simulink model "sim_battery"  (R2022b)
settings: Solver=VariableStepAuto  StartTime=0.0  StopTime=2001  RelTol=1e-3
undefined symbols (not defined in the file or in its folder): battery_builder_rtmsupport, gcbh
libraries: nesl_utility x14, GD_Batterymodel_5_lib x8, fl_lib x7, BatteryCurrentManagement x1, batt_lib x1, BatteryBalancing x1, simulink x1, SimscapeFluids_lib x1
(part 2 of 2)

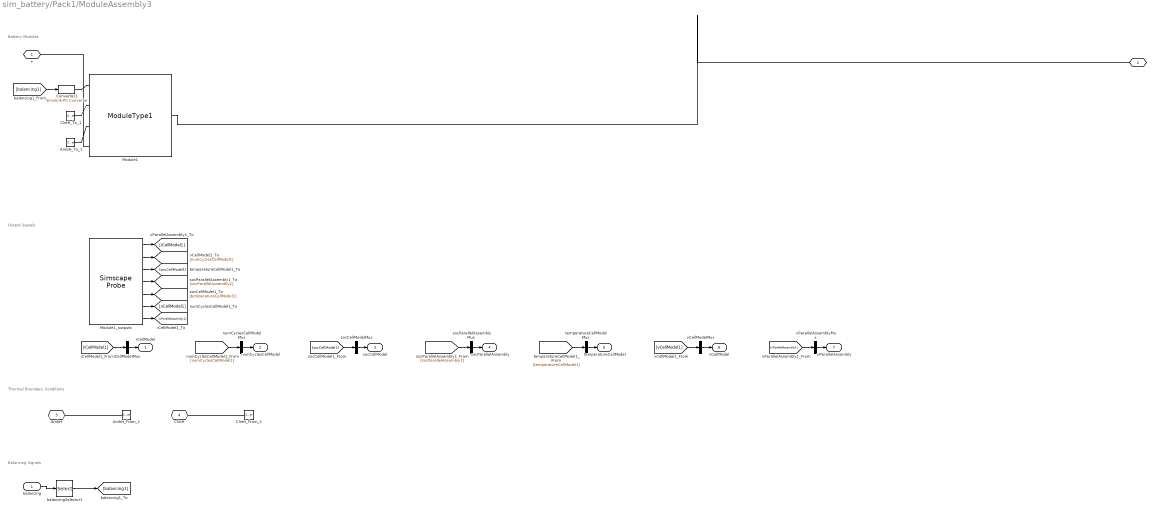
== system sim_battery/Pack1/ModuleAssembly3 ==
  note: Balancing Signals
  note: Thermal Boundary Conditions
  note: Output Signals
  note: Battery Modules
  balancing : Inport  PortDimensions=14
  AmbH_From_1 : ConnectionLabel  Label=ambH_1
  AmbH_To_1 : ConnectionLabel  Label=ambH_1
  ClntH_From_1 : ConnectionLabel  Label=clntH_1
  ClntH_To_1 : ConnectionLabel  Label=clntH_1
  Converter1 : nesl_utility/Simulink-PS Converter  PhysicalDomain=network_engine_domain  SubClassName=ps_input  LeftPortType=input  RightPortType=output  PseudoPeriodic=off  Frequencies=[]  NoiseDistribution=none  NoiseParameters=[]  Unit=1  AffineConversion=off  FilteringAndDerivatives=provide  SimscapeFilterOrder=1  InputFilterTimeConstant=0.001  UdotUserProvided=0
  Module1 : GD_Batterymodel_5_lib/Modules/ModuleType1  SOC_vec=ModuleType1.SOC_vec  T_vec=ModuleType1.T_vec K  V0_mat=ModuleType1.V0_mat V  V_range=ModuleType1.V_range V  R0_mat=ModuleType1.R0_mat Ohm  AH=ModuleType1.AH A*hr  extrapolation_option=simscape.enum.extrapolation.nearest  R1_mat=ModuleType1.R1_mat Ohm  tau1_mat=ModuleType1.tau1_mat s  R2_mat=ModuleType1.R2_mat Ohm  tau2_mat=ModuleType1.tau2_mat s  thermal_mass=ModuleType1.thermal_mass J/K  CoolantResistance=ModuleType1.CoolantResistance K/W  AmbientResistance=ModuleType1.AmbientResistance K/W  CellBalancingClosedResistance=ModuleType1.CellBalancingClosedResistance Ohm  CellBalancingOpenConductance=ModuleType1.CellBalancingOpenConductance 1/Ohm  CellBalancingThreshold=ModuleType1.CellBalancingThreshold  CellBalancingResistance=ModuleType1.CellBalancingResistance Ohm  P=3  S=14  iCellModel_specify=on  iCellModel_priority=None  iCellModel=ModuleAssembly3.Module1.iCellModel A  iCellModel_nominal_specify=off  iCellModel_nominal_unit=A  iCellModel_nominal_value=1  vCellModel_specify=on  vCellModel_priority=None  vCellModel=ModuleAssembly3.Module1.vCellModel V  vCellModel_nominal_specify=off  vCellModel_nominal_unit=V  vCellModel_nominal_value=1  socCellModel_specify=on  socCellModel_priority=High  socCellModel=ModuleAssembly3.Module1.socCellModel  socCellModel_nominal_specify=off  socCellModel_nominal_unit=1  socCellModel_nominal_value=1  numCyclesCellModel_specify=on  numCyclesCellModel_priority=High  numCyclesCellModel=ModuleAssembly3.Module1.numCyclesCellModel  numCyclesCellModel_nominal_specify=off  numCyclesCellModel_nominal_unit=1  numCyclesCellModel_nominal_value=1  temperatureCellModel_specify=on  temperatureCellModel_priority=High  temperatureCellModel=ModuleAssembly3.Module1.temperatureCellModel K  temperatureCellModel_nominal_specify=off  temperatureCellModel_nominal_unit=K  temperatureCellModel_nominal_value=1  vParallelAssembly_specify=on  vParallelAssembly_priority=None  vParallelAssembly=ModuleAssembly3.Module1.vParallelAssembly V  vParallelAssembly_nominal_specify=off  vParallelAssembly_nominal_unit=V  vParallelAssembly_nominal_value=1  socParallelAssembly_specify=on  socParallelAssembly_priority=None  socParallelAssembly=ModuleAssembly3.Module1.socParallelAssembly  socParallelAssembly_nominal_specify=off  socParallelAssembly_nominal_unit=1  socParallelAssembly_nominal_value=1
      settings: InternalSimscapePortConfiguration="{\"Bottom\":[{\"id\":\"n\",\"label\":\"-\",\"type\":\"foundation.electrical.electrical\"}],\"Left\":[{\"id\":\"enableCellBalancing\",\"label\":\"CB\",\"type\":\"input\"},{\"id\":\"ClntH\",\"label\":\"CH\",\"type\":\"foundation.thermal.thermal\"},{\"id\":\"AmbH\",\"label\":\"AH\",\"type\":\"foundation.thermal.thermal\"}],\"Right\":[],\"Top\":[{\"id\":\"p\",\"label\":\"+\",\"type\":\"foundation.electrical.electrical\"}]}"
  Module1_outputs : SimscapeProbe  BoundBlock=1476  Variables={iCellModel, numCyclesCellModel, socCellModel, socParallelAssembly, temperatureCellModel, vCellModel, vParallelAssembly}
  balancingSelector1 : Selector  InputPortWidth=14  IndexOptions=Index vector (dialog)  Indices="[1   2   3   4   5   6   7   8   9  10  11  12  13  14]"  OutputSizes=1
  iCellModelMux : Mux  Inputs=1
  numCyclesCellModelMux : Mux  Inputs=1
  socCellModelMux : Mux  Inputs=1
  socParallelAssemblyMux : Mux  Inputs=1
  temperatureCellModelMux : Mux  Inputs=1
  vCellModelMux : Mux  Inputs=1
  vParallelAssemblyMux : Mux  Inputs=1
  + : PMIOPort  Side=Left
  - : PMIOPort  Port=2  Side=Right
  AmbH : PMIOPort  Port=3  Side=Right
  ClntH : PMIOPort  Port=4  Side=Right
  iCellModel : Outport
  numCyclesCellModel : Outport  Port=2
  socCellModel : Outport  Port=3
  socParallelAssembly : Outport  Port=4
  temperatureCellModel : Outport  Port=5
  vCellModel : Outport  Port=6
  vParallelAssembly : Outport  Port=7
  wires:
  [balancing1] -> Converter1/1
  balancingSelector1/1 -> [balancing1]
  balancing/1 -> balancingSelector1/1
  [vParallelAssembly1] -> vParallelAssemblyMux/1
  vParallelAssemblyMux/1 -> vParallelAssembly/1
  Module1_outputs/1 -> [iCellModel1]
  [vCellModel1] -> vCellModelMux/1
  vCellModelMux/1 -> vCellModel/1
  Module1_outputs/2 -> [numCyclesCellModel1]
  [temperatureCellModel1] -> temperatureCellModelMux/1
  temperatureCellModelMux/1 -> temperatureCellModel/1
  Module1_outputs/3 -> [socCellModel1]
  [socParallelAssembly1] -> socParallelAssemblyMux/1
  socParallelAssemblyMux/1 -> socParallelAssembly/1
  Module1_outputs/4 -> [socParallelAssembly1]
  [socCellModel1] -> socCellModelMux/1
  socCellModelMux/1 -> socCellModel/1
  Module1_outputs/5 -> [temperatureCellModel1]
  [numCyclesCellModel1] -> numCyclesCellModelMux/1
  numCyclesCellModelMux/1 -> numCyclesCellModel/1
  Module1_outputs/6 -> [vCellModel1]
  [iCellModel1] -> iCellModelMux/1
  iCellModelMux/1 -> iCellModel/1
  Module1_outputs/7 -> [vParallelAssembly1]
  connections:
  Converter1/RConn1 -- Module1/LConn1
  ClntH_From_1/LConn1 -- ClntH/RConn1
  ClntH_To_1/LConn1 -- Module1/LConn2
  AmbH_From_1/LConn1 -- AmbH/RConn1
  AmbH_To_1/LConn1 -- Module1/LConn3
  Module1/RConn1 -- -/RConn1
  Module1/LConn4 -- +/RConn1

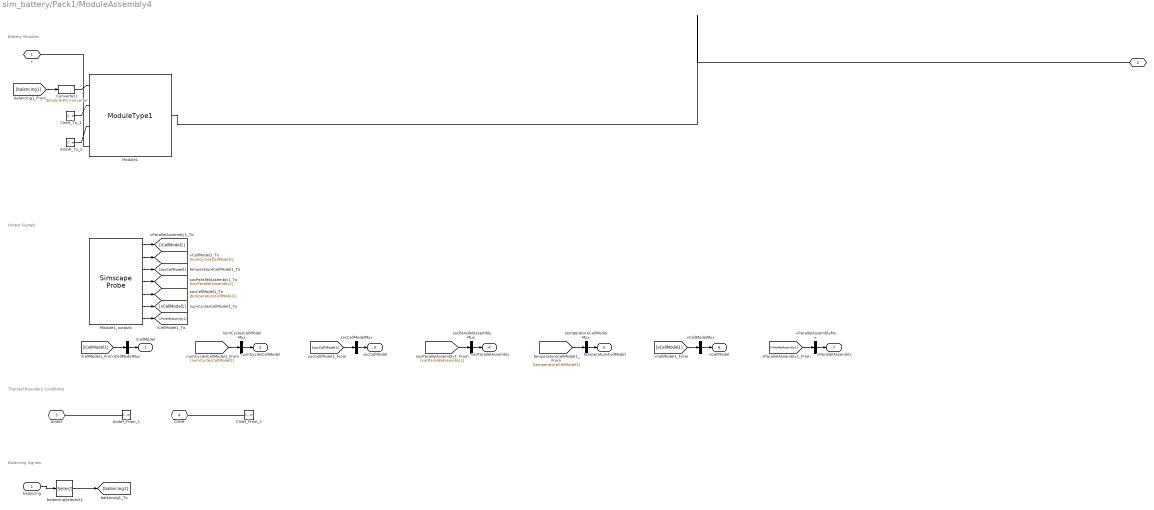
== system sim_battery/Pack1/ModuleAssembly4 ==
  note: Balancing Signals
  note: Thermal Boundary Conditions
  note: Output Signals
  note: Battery Modules
  balancing : Inport  PortDimensions=14
  AmbH_From_1 : ConnectionLabel  Label=ambH_1
  AmbH_To_1 : ConnectionLabel  Label=ambH_1
  ClntH_From_1 : ConnectionLabel  Label=clntH_1
  ClntH_To_1 : ConnectionLabel  Label=clntH_1
  Converter1 : nesl_utility/Simulink-PS Converter  PhysicalDomain=network_engine_domain  SubClassName=ps_input  LeftPortType=input  RightPortType=output  PseudoPeriodic=off  Frequencies=[]  NoiseDistribution=none  NoiseParameters=[]  Unit=1  AffineConversion=off  FilteringAndDerivatives=provide  SimscapeFilterOrder=1  InputFilterTimeConstant=0.001  UdotUserProvided=0
  Module1 : GD_Batterymodel_5_lib/Modules/ModuleType1  SOC_vec=ModuleType1.SOC_vec  T_vec=ModuleType1.T_vec K  V0_mat=ModuleType1.V0_mat V  V_range=ModuleType1.V_range V  R0_mat=ModuleType1.R0_mat Ohm  AH=ModuleType1.AH A*hr  extrapolation_option=simscape.enum.extrapolation.nearest  R1_mat=ModuleType1.R1_mat Ohm  tau1_mat=ModuleType1.tau1_mat s  R2_mat=ModuleType1.R2_mat Ohm  tau2_mat=ModuleType1.tau2_mat s  thermal_mass=ModuleType1.thermal_mass J/K  CoolantResistance=ModuleType1.CoolantResistance K/W  AmbientResistance=ModuleType1.AmbientResistance K/W  CellBalancingClosedResistance=ModuleType1.CellBalancingClosedResistance Ohm  CellBalancingOpenConductance=ModuleType1.CellBalancingOpenConductance 1/Ohm  CellBalancingThreshold=ModuleType1.CellBalancingThreshold  CellBalancingResistance=ModuleType1.CellBalancingResistance Ohm  P=3  S=14  iCellModel_specify=on  iCellModel_priority=None  iCellModel=ModuleAssembly4.Module1.iCellModel A  iCellModel_nominal_specify=off  iCellModel_nominal_unit=A  iCellModel_nominal_value=1  vCellModel_specify=on  vCellModel_priority=None  vCellModel=ModuleAssembly4.Module1.vCellModel V  vCellModel_nominal_specify=off  vCellModel_nominal_unit=V  vCellModel_nominal_value=1  socCellModel_specify=on  socCellModel_priority=High  socCellModel=ModuleAssembly4.Module1.socCellModel  socCellModel_nominal_specify=off  socCellModel_nominal_unit=1  socCellModel_nominal_value=1  numCyclesCellModel_specify=on  numCyclesCellModel_priority=High  numCyclesCellModel=ModuleAssembly4.Module1.numCyclesCellModel  numCyclesCellModel_nominal_specify=off  numCyclesCellModel_nominal_unit=1  numCyclesCellModel_nominal_value=1  temperatureCellModel_specify=on  temperatureCellModel_priority=High  temperatureCellModel=ModuleAssembly4.Module1.temperatureCellModel K  temperatureCellModel_nominal_specify=off  temperatureCellModel_nominal_unit=K  temperatureCellModel_nominal_value=1  vParallelAssembly_specify=on  vParallelAssembly_priority=None  vParallelAssembly=ModuleAssembly4.Module1.vParallelAssembly V  vParallelAssembly_nominal_specify=off  vParallelAssembly_nominal_unit=V  vParallelAssembly_nominal_value=1  socParallelAssembly_specify=on  socParallelAssembly_priority=None  socParallelAssembly=ModuleAssembly4.Module1.socParallelAssembly  socParallelAssembly_nominal_specify=off  socParallelAssembly_nominal_unit=1  socParallelAssembly_nominal_value=1
      settings: InternalSimscapePortConfiguration="{\"Bottom\":[{\"id\":\"n\",\"label\":\"-\",\"type\":\"foundation.electrical.electrical\"}],\"Left\":[{\"id\":\"enableCellBalancing\",\"label\":\"CB\",\"type\":\"input\"},{\"id\":\"ClntH\",\"label\":\"CH\",\"type\":\"foundation.thermal.thermal\"},{\"id\":\"AmbH\",\"label\":\"AH\",\"type\":\"foundation.thermal.thermal\"}],\"Right\":[],\"Top\":[{\"id\":\"p\",\"label\":\"+\",\"type\":\"foundation.electrical.electrical\"}]}"
  Module1_outputs : SimscapeProbe  BoundBlock=1524  Variables={iCellModel, numCyclesCellModel, socCellModel, socParallelAssembly, temperatureCellModel, vCellModel, vParallelAssembly}
  balancingSelector1 : Selector  InputPortWidth=14  IndexOptions=Index vector (dialog)  Indices="[1   2   3   4   5   6   7   8   9  10  11  12  13  14]"  OutputSizes=1
  iCellModelMux : Mux  Inputs=1
  numCyclesCellModelMux : Mux  Inputs=1
  socCellModelMux : Mux  Inputs=1
  socParallelAssemblyMux : Mux  Inputs=1
  temperatureCellModelMux : Mux  Inputs=1
  vCellModelMux : Mux  Inputs=1
  vParallelAssemblyMux : Mux  Inputs=1
  + : PMIOPort  Side=Left
  - : PMIOPort  Port=2  Side=Right
  AmbH : PMIOPort  Port=3  Side=Right
  ClntH : PMIOPort  Port=4  Side=Right
  iCellModel : Outport
  numCyclesCellModel : Outport  Port=2
  socCellModel : Outport  Port=3
  socParallelAssembly : Outport  Port=4
  temperatureCellModel : Outport  Port=5
  vCellModel : Outport  Port=6
  vParallelAssembly : Outport  Port=7
  wires:
  [balancing1] -> Converter1/1
  balancingSelector1/1 -> [balancing1]
  balancing/1 -> balancingSelector1/1
  [vParallelAssembly1] -> vParallelAssemblyMux/1
  vParallelAssemblyMux/1 -> vParallelAssembly/1
  Module1_outputs/1 -> [iCellModel1]
  [vCellModel1] -> vCellModelMux/1
  vCellModelMux/1 -> vCellModel/1
  Module1_outputs/2 -> [numCyclesCellModel1]
  [temperatureCellModel1] -> temperatureCellModelMux/1
  temperatureCellModelMux/1 -> temperatureCellModel/1
  Module1_outputs/3 -> [socCellModel1]
  [socParallelAssembly1] -> socParallelAssemblyMux/1
  socParallelAssemblyMux/1 -> socParallelAssembly/1
  Module1_outputs/4 -> [socParallelAssembly1]
  [socCellModel1] -> socCellModelMux/1
  socCellModelMux/1 -> socCellModel/1
  Module1_outputs/5 -> [temperatureCellModel1]
  [numCyclesCellModel1] -> numCyclesCellModelMux/1
  numCyclesCellModelMux/1 -> numCyclesCellModel/1
  Module1_outputs/6 -> [vCellModel1]
  [iCellModel1] -> iCellModelMux/1
  iCellModelMux/1 -> iCellModel/1
  Module1_outputs/7 -> [vParallelAssembly1]
  connections:
  Converter1/RConn1 -- Module1/LConn1
  ClntH_From_1/LConn1 -- ClntH/RConn1
  ClntH_To_1/LConn1 -- Module1/LConn2
  AmbH_From_1/LConn1 -- AmbH/RConn1
  AmbH_To_1/LConn1 -- Module1/LConn3
  Module1/RConn1 -- -/RConn1
  Module1/LConn4 -- +/RConn1

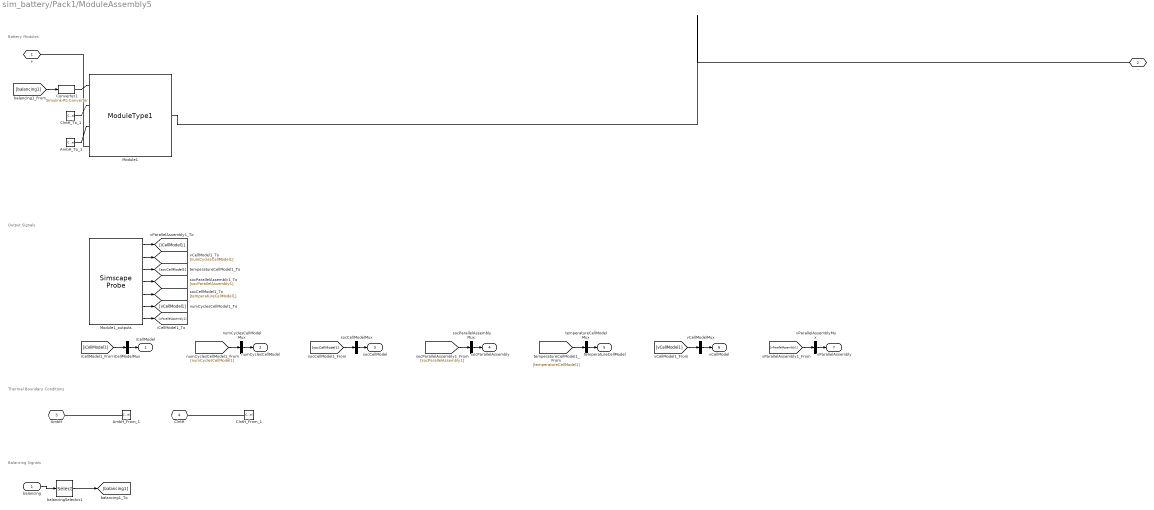
== system sim_battery/Pack1/ModuleAssembly5 ==
  note: Balancing Signals
  note: Thermal Boundary Conditions
  note: Output Signals
  note: Battery Modules
  balancing : Inport  PortDimensions=14
  AmbH_From_1 : ConnectionLabel  Label=ambH_1
  AmbH_To_1 : ConnectionLabel  Label=ambH_1
  ClntH_From_1 : ConnectionLabel  Label=clntH_1
  ClntH_To_1 : ConnectionLabel  Label=clntH_1
  Converter1 : nesl_utility/Simulink-PS Converter  PhysicalDomain=network_engine_domain  SubClassName=ps_input  LeftPortType=input  RightPortType=output  PseudoPeriodic=off  Frequencies=[]  NoiseDistribution=none  NoiseParameters=[]  Unit=1  AffineConversion=off  FilteringAndDerivatives=provide  SimscapeFilterOrder=1  InputFilterTimeConstant=0.001  UdotUserProvided=0
  Module1 : GD_Batterymodel_5_lib/Modules/ModuleType1  SOC_vec=ModuleType1.SOC_vec  T_vec=ModuleType1.T_vec K  V0_mat=ModuleType1.V0_mat V  V_range=ModuleType1.V_range V  R0_mat=ModuleType1.R0_mat Ohm  AH=ModuleType1.AH A*hr  extrapolation_option=simscape.enum.extrapolation.nearest  R1_mat=ModuleType1.R1_mat Ohm  tau1_mat=ModuleType1.tau1_mat s  R2_mat=ModuleType1.R2_mat Ohm  tau2_mat=ModuleType1.tau2_mat s  thermal_mass=ModuleType1.thermal_mass J/K  CoolantResistance=ModuleType1.CoolantResistance K/W  AmbientResistance=ModuleType1.AmbientResistance K/W  CellBalancingClosedResistance=ModuleType1.CellBalancingClosedResistance Ohm  CellBalancingOpenConductance=ModuleType1.CellBalancingOpenConductance 1/Ohm  CellBalancingThreshold=ModuleType1.CellBalancingThreshold  CellBalancingResistance=ModuleType1.CellBalancingResistance Ohm  P=3  S=14  iCellModel_specify=on  iCellModel_priority=None  iCellModel=ModuleAssembly5.Module1.iCellModel A  iCellModel_nominal_specify=off  iCellModel_nominal_unit=A  iCellModel_nominal_value=1  vCellModel_specify=on  vCellModel_priority=None  vCellModel=ModuleAssembly5.Module1.vCellModel V  vCellModel_nominal_specify=off  vCellModel_nominal_unit=V  vCellModel_nominal_value=1  socCellModel_specify=on  socCellModel_priority=High  socCellModel=ModuleAssembly5.Module1.socCellModel  socCellModel_nominal_specify=off  socCellModel_nominal_unit=1  socCellModel_nominal_value=1  numCyclesCellModel_specify=on  numCyclesCellModel_priority=High  numCyclesCellModel=ModuleAssembly5.Module1.numCyclesCellModel  numCyclesCellModel_nominal_specify=off  numCyclesCellModel_nominal_unit=1  numCyclesCellModel_nominal_value=1  temperatureCellModel_specify=on  temperatureCellModel_priority=High  temperatureCellModel=ModuleAssembly5.Module1.temperatureCellModel K  temperatureCellModel_nominal_specify=off  temperatureCellModel_nominal_unit=K  temperatureCellModel_nominal_value=1  vParallelAssembly_specify=on  vParallelAssembly_priority=None  vParallelAssembly=ModuleAssembly5.Module1.vParallelAssembly V  vParallelAssembly_nominal_specify=off  vParallelAssembly_nominal_unit=V  vParallelAssembly_nominal_value=1  socParallelAssembly_specify=on  socParallelAssembly_priority=None  socParallelAssembly=ModuleAssembly5.Module1.socParallelAssembly  socParallelAssembly_nominal_specify=off  socParallelAssembly_nominal_unit=1  socParallelAssembly_nominal_value=1
      settings: InternalSimscapePortConfiguration="{\"Bottom\":[{\"id\":\"n\",\"label\":\"-\",\"type\":\"foundation.electrical.electrical\"}],\"Left\":[{\"id\":\"enableCellBalancing\",\"label\":\"CB\",\"type\":\"input\"},{\"id\":\"ClntH\",\"label\":\"CH\",\"type\":\"foundation.thermal.thermal\"},{\"id\":\"AmbH\",\"label\":\"AH\",\"type\":\"foundation.thermal.thermal\"}],\"Right\":[],\"Top\":[{\"id\":\"p\",\"label\":\"+\",\"type\":\"foundation.electrical.electrical\"}]}"
  Module1_outputs : SimscapeProbe  BoundBlock=1572  Variables={iCellModel, numCyclesCellModel, socCellModel, socParallelAssembly, temperatureCellModel, vCellModel, vParallelAssembly}
  balancingSelector1 : Selector  InputPortWidth=14  IndexOptions=Index vector (dialog)  Indices="[1   2   3   4   5   6   7   8   9  10  11  12  13  14]"  OutputSizes=1
  iCellModelMux : Mux  Inputs=1
  numCyclesCellModelMux : Mux  Inputs=1
  socCellModelMux : Mux  Inputs=1
  socParallelAssemblyMux : Mux  Inputs=1
  temperatureCellModelMux : Mux  Inputs=1
  vCellModelMux : Mux  Inputs=1
  vParallelAssemblyMux : Mux  Inputs=1
  + : PMIOPort  Side=Left
  - : PMIOPort  Port=2  Side=Right
  AmbH : PMIOPort  Port=3  Side=Right
  ClntH : PMIOPort  Port=4  Side=Right
  iCellModel : Outport
  numCyclesCellModel : Outport  Port=2
  socCellModel : Outport  Port=3
  socParallelAssembly : Outport  Port=4
  temperatureCellModel : Outport  Port=5
  vCellModel : Outport  Port=6
  vParallelAssembly : Outport  Port=7
  wires:
  [balancing1] -> Converter1/1
  balancingSelector1/1 -> [balancing1]
  balancing/1 -> balancingSelector1/1
  [vParallelAssembly1] -> vParallelAssemblyMux/1
  vParallelAssemblyMux/1 -> vParallelAssembly/1
  Module1_outputs/1 -> [iCellModel1]
  [vCellModel1] -> vCellModelMux/1
  vCellModelMux/1 -> vCellModel/1
  Module1_outputs/2 -> [numCyclesCellModel1]
  [temperatureCellModel1] -> temperatureCellModelMux/1
  temperatureCellModelMux/1 -> temperatureCellModel/1
  Module1_outputs/3 -> [socCellModel1]
  [socParallelAssembly1] -> socParallelAssemblyMux/1
  socParallelAssemblyMux/1 -> socParallelAssembly/1
  Module1_outputs/4 -> [socParallelAssembly1]
  [socCellModel1] -> socCellModelMux/1
  socCellModelMux/1 -> socCellModel/1
  Module1_outputs/5 -> [temperatureCellModel1]
  [numCyclesCellModel1] -> numCyclesCellModelMux/1
  numCyclesCellModelMux/1 -> numCyclesCellModel/1
  Module1_outputs/6 -> [vCellModel1]
  [iCellModel1] -> iCellModelMux/1
  iCellModelMux/1 -> iCellModel/1
  Module1_outputs/7 -> [vParallelAssembly1]
  connections:
  Converter1/RConn1 -- Module1/LConn1
  ClntH_From_1/LConn1 -- ClntH/RConn1
  ClntH_To_1/LConn1 -- Module1/LConn2
  AmbH_From_1/LConn1 -- AmbH/RConn1
  AmbH_To_1/LConn1 -- Module1/LConn3
  Module1/RConn1 -- -/RConn1
  Module1/LConn4 -- +/RConn1

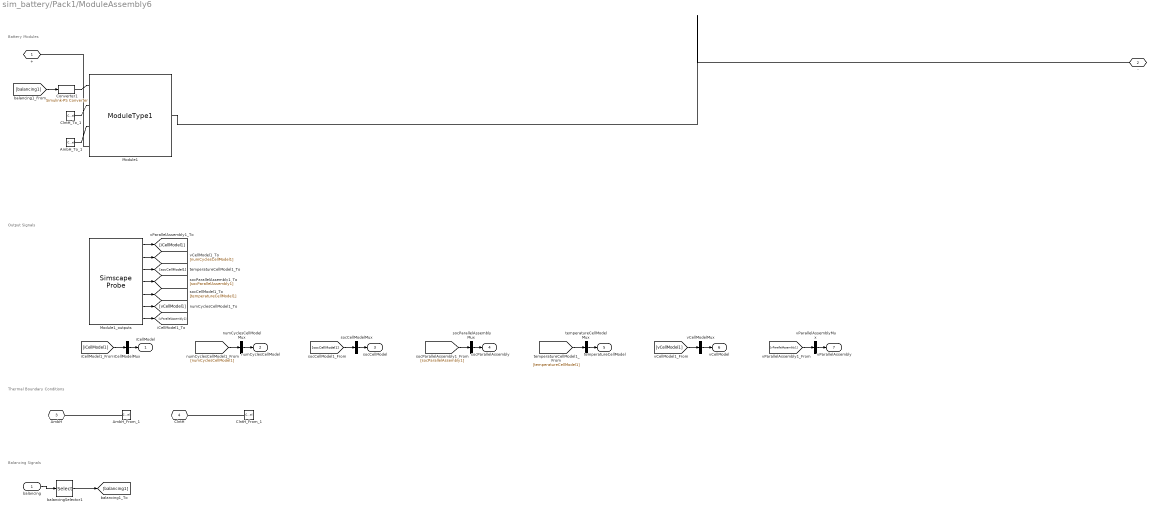
== system sim_battery/Pack1/ModuleAssembly6 ==
  note: Balancing Signals
  note: Thermal Boundary Conditions
  note: Output Signals
  note: Battery Modules
  balancing : Inport  PortDimensions=14
  AmbH_From_1 : ConnectionLabel  Label=ambH_1
  AmbH_To_1 : ConnectionLabel  Label=ambH_1
  ClntH_From_1 : ConnectionLabel  Label=clntH_1
  ClntH_To_1 : ConnectionLabel  Label=clntH_1
  Converter1 : nesl_utility/Simulink-PS Converter  PhysicalDomain=network_engine_domain  SubClassName=ps_input  LeftPortType=input  RightPortType=output  PseudoPeriodic=off  Frequencies=[]  NoiseDistribution=none  NoiseParameters=[]  Unit=1  AffineConversion=off  FilteringAndDerivatives=provide  SimscapeFilterOrder=1  InputFilterTimeConstant=0.001  UdotUserProvided=0
  Module1 : GD_Batterymodel_5_lib/Modules/ModuleType1  SOC_vec=ModuleType1.SOC_vec  T_vec=ModuleType1.T_vec K  V0_mat=ModuleType1.V0_mat V  V_range=ModuleType1.V_range V  R0_mat=ModuleType1.R0_mat Ohm  AH=ModuleType1.AH A*hr  extrapolation_option=simscape.enum.extrapolation.nearest  R1_mat=ModuleType1.R1_mat Ohm  tau1_mat=ModuleType1.tau1_mat s  R2_mat=ModuleType1.R2_mat Ohm  tau2_mat=ModuleType1.tau2_mat s  thermal_mass=ModuleType1.thermal_mass J/K  CoolantResistance=ModuleType1.CoolantResistance K/W  AmbientResistance=ModuleType1.AmbientResistance K/W  CellBalancingClosedResistance=ModuleType1.CellBalancingClosedResistance Ohm  CellBalancingOpenConductance=ModuleType1.CellBalancingOpenConductance 1/Ohm  CellBalancingThreshold=ModuleType1.CellBalancingThreshold  CellBalancingResistance=ModuleType1.CellBalancingResistance Ohm  P=3  S=14  iCellModel_specify=on  iCellModel_priority=None  iCellModel=ModuleAssembly6.Module1.iCellModel A  iCellModel_nominal_specify=off  iCellModel_nominal_unit=A  iCellModel_nominal_value=1  vCellModel_specify=on  vCellModel_priority=None  vCellModel=ModuleAssembly6.Module1.vCellModel V  vCellModel_nominal_specify=off  vCellModel_nominal_unit=V  vCellModel_nominal_value=1  socCellModel_specify=on  socCellModel_priority=High  socCellModel=ModuleAssembly6.Module1.socCellModel  socCellModel_nominal_specify=off  socCellModel_nominal_unit=1  socCellModel_nominal_value=1  numCyclesCellModel_specify=on  numCyclesCellModel_priority=High  numCyclesCellModel=ModuleAssembly6.Module1.numCyclesCellModel  numCyclesCellModel_nominal_specify=off  numCyclesCellModel_nominal_unit=1  numCyclesCellModel_nominal_value=1  temperatureCellModel_specify=on  temperatureCellModel_priority=High  temperatureCellModel=ModuleAssembly6.Module1.temperatureCellModel K  temperatureCellModel_nominal_specify=off  temperatureCellModel_nominal_unit=K  temperatureCellModel_nominal_value=1  vParallelAssembly_specify=on  vParallelAssembly_priority=None  vParallelAssembly=ModuleAssembly6.Module1.vParallelAssembly V  vParallelAssembly_nominal_specify=off  vParallelAssembly_nominal_unit=V  vParallelAssembly_nominal_value=1  socParallelAssembly_specify=on  socParallelAssembly_priority=None  socParallelAssembly=ModuleAssembly6.Module1.socParallelAssembly  socParallelAssembly_nominal_specify=off  socParallelAssembly_nominal_unit=1  socParallelAssembly_nominal_value=1
      settings: InternalSimscapePortConfiguration="{\"Bottom\":[{\"id\":\"n\",\"label\":\"-\",\"type\":\"foundation.electrical.electrical\"}],\"Left\":[{\"id\":\"enableCellBalancing\",\"label\":\"CB\",\"type\":\"input\"},{\"id\":\"ClntH\",\"label\":\"CH\",\"type\":\"foundation.thermal.thermal\"},{\"id\":\"AmbH\",\"label\":\"AH\",\"type\":\"foundation.thermal.thermal\"}],\"Right\":[],\"Top\":[{\"id\":\"p\",\"label\":\"+\",\"type\":\"foundation.electrical.electrical\"}]}"
  Module1_outputs : SimscapeProbe  BoundBlock=1620  Variables={iCellModel, numCyclesCellModel, socCellModel, socParallelAssembly, temperatureCellModel, vCellModel, vParallelAssembly}
  balancingSelector1 : Selector  InputPortWidth=14  IndexOptions=Index vector (dialog)  Indices="[1   2   3   4   5   6   7   8   9  10  11  12  13  14]"  OutputSizes=1
  iCellModelMux : Mux  Inputs=1
  numCyclesCellModelMux : Mux  Inputs=1
  socCellModelMux : Mux  Inputs=1
  socParallelAssemblyMux : Mux  Inputs=1
  temperatureCellModelMux : Mux  Inputs=1
  vCellModelMux : Mux  Inputs=1
  vParallelAssemblyMux : Mux  Inputs=1
  + : PMIOPort  Side=Left
  - : PMIOPort  Port=2  Side=Right
  AmbH : PMIOPort  Port=3  Side=Right
  ClntH : PMIOPort  Port=4  Side=Right
  iCellModel : Outport
  numCyclesCellModel : Outport  Port=2
  socCellModel : Outport  Port=3
  socParallelAssembly : Outport  Port=4
  temperatureCellModel : Outport  Port=5
  vCellModel : Outport  Port=6
  vParallelAssembly : Outport  Port=7
  wires:
  [balancing1] -> Converter1/1
  balancingSelector1/1 -> [balancing1]
  balancing/1 -> balancingSelector1/1
  [vParallelAssembly1] -> vParallelAssemblyMux/1
  vParallelAssemblyMux/1 -> vParallelAssembly/1
  Module1_outputs/1 -> [iCellModel1]
  [vCellModel1] -> vCellModelMux/1
  vCellModelMux/1 -> vCellModel/1
  Module1_outputs/2 -> [numCyclesCellModel1]
  [temperatureCellModel1] -> temperatureCellModelMux/1
  temperatureCellModelMux/1 -> temperatureCellModel/1
  Module1_outputs/3 -> [socCellModel1]
  [socParallelAssembly1] -> socParallelAssemblyMux/1
  socParallelAssemblyMux/1 -> socParallelAssembly/1
  Module1_outputs/4 -> [socParallelAssembly1]
  [socCellModel1] -> socCellModelMux/1
  socCellModelMux/1 -> socCellModel/1
  Module1_outputs/5 -> [temperatureCellModel1]
  [numCyclesCellModel1] -> numCyclesCellModelMux/1
  numCyclesCellModelMux/1 -> numCyclesCellModel/1
  Module1_outputs/6 -> [vCellModel1]
  [iCellModel1] -> iCellModelMux/1
  iCellModelMux/1 -> iCellModel/1
  Module1_outputs/7 -> [vParallelAssembly1]
  connections:
  Converter1/RConn1 -- Module1/LConn1
  ClntH_From_1/LConn1 -- ClntH/RConn1
  ClntH_To_1/LConn1 -- Module1/LConn2
  AmbH_From_1/LConn1 -- AmbH/RConn1
  AmbH_To_1/LConn1 -- Module1/LConn3
  Module1/RConn1 -- -/RConn1
  Module1/LConn4 -- +/RConn1

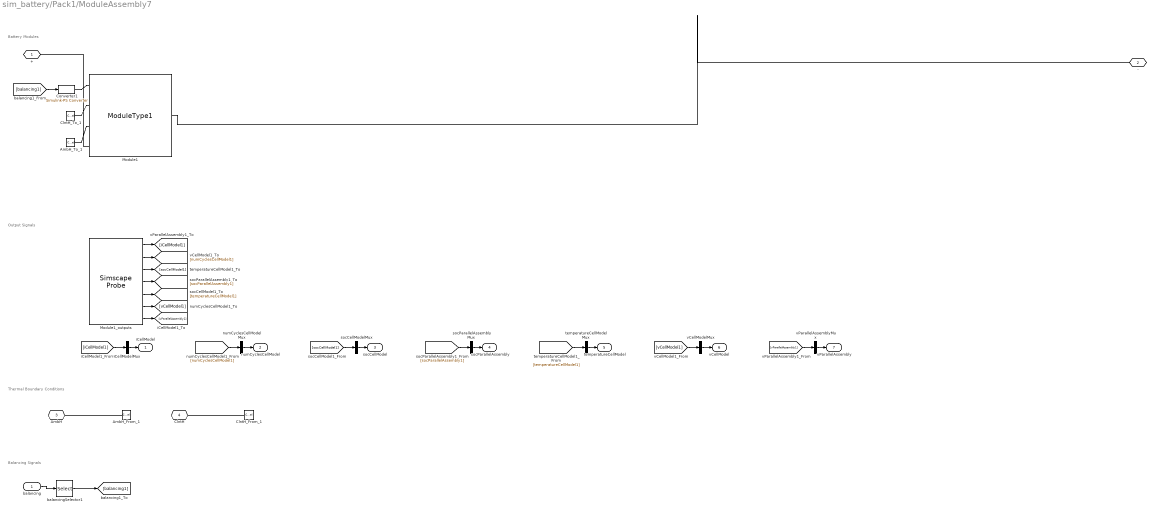
== system sim_battery/Pack1/ModuleAssembly7 ==
  note: Balancing Signals
  note: Thermal Boundary Conditions
  note: Output Signals
  note: Battery Modules
  balancing : Inport  PortDimensions=14
  AmbH_From_1 : ConnectionLabel  Label=ambH_1
  AmbH_To_1 : ConnectionLabel  Label=ambH_1
  ClntH_From_1 : ConnectionLabel  Label=clntH_1
  ClntH_To_1 : ConnectionLabel  Label=clntH_1
  Converter1 : nesl_utility/Simulink-PS Converter  PhysicalDomain=network_engine_domain  SubClassName=ps_input  LeftPortType=input  RightPortType=output  PseudoPeriodic=off  Frequencies=[]  NoiseDistribution=none  NoiseParameters=[]  Unit=1  AffineConversion=off  FilteringAndDerivatives=provide  SimscapeFilterOrder=1  InputFilterTimeConstant=0.001  UdotUserProvided=0
  Module1 : GD_Batterymodel_5_lib/Modules/ModuleType1  SOC_vec=ModuleType1.SOC_vec  T_vec=ModuleType1.T_vec K  V0_mat=ModuleType1.V0_mat V  V_range=ModuleType1.V_range V  R0_mat=ModuleType1.R0_mat Ohm  AH=ModuleType1.AH A*hr  extrapolation_option=simscape.enum.extrapolation.nearest  R1_mat=ModuleType1.R1_mat Ohm  tau1_mat=ModuleType1.tau1_mat s  R2_mat=ModuleType1.R2_mat Ohm  tau2_mat=ModuleType1.tau2_mat s  thermal_mass=ModuleType1.thermal_mass J/K  CoolantResistance=ModuleType1.CoolantResistance K/W  AmbientResistance=ModuleType1.AmbientResistance K/W  CellBalancingClosedResistance=ModuleType1.CellBalancingClosedResistance Ohm  CellBalancingOpenConductance=ModuleType1.CellBalancingOpenConductance 1/Ohm  CellBalancingThreshold=ModuleType1.CellBalancingThreshold  CellBalancingResistance=ModuleType1.CellBalancingResistance Ohm  P=3  S=14  iCellModel_specify=on  iCellModel_priority=None  iCellModel=ModuleAssembly7.Module1.iCellModel A  iCellModel_nominal_specify=off  iCellModel_nominal_unit=A  iCellModel_nominal_value=1  vCellModel_specify=on  vCellModel_priority=None  vCellModel=ModuleAssembly7.Module1.vCellModel V  vCellModel_nominal_specify=off  vCellModel_nominal_unit=V  vCellModel_nominal_value=1  socCellModel_specify=on  socCellModel_priority=High  socCellModel=ModuleAssembly7.Module1.socCellModel  socCellModel_nominal_specify=off  socCellModel_nominal_unit=1  socCellModel_nominal_value=1  numCyclesCellModel_specify=on  numCyclesCellModel_priority=High  numCyclesCellModel=ModuleAssembly7.Module1.numCyclesCellModel  numCyclesCellModel_nominal_specify=off  numCyclesCellModel_nominal_unit=1  numCyclesCellModel_nominal_value=1  temperatureCellModel_specify=on  temperatureCellModel_priority=High  temperatureCellModel=ModuleAssembly7.Module1.temperatureCellModel K  temperatureCellModel_nominal_specify=off  temperatureCellModel_nominal_unit=K  temperatureCellModel_nominal_value=1  vParallelAssembly_specify=on  vParallelAssembly_priority=None  vParallelAssembly=ModuleAssembly7.Module1.vParallelAssembly V  vParallelAssembly_nominal_specify=off  vParallelAssembly_nominal_unit=V  vParallelAssembly_nominal_value=1  socParallelAssembly_specify=on  socParallelAssembly_priority=None  socParallelAssembly=ModuleAssembly7.Module1.socParallelAssembly  socParallelAssembly_nominal_specify=off  socParallelAssembly_nominal_unit=1  socParallelAssembly_nominal_value=1
      settings: InternalSimscapePortConfiguration="{\"Bottom\":[{\"id\":\"n\",\"label\":\"-\",\"type\":\"foundation.electrical.electrical\"}],\"Left\":[{\"id\":\"enableCellBalancing\",\"label\":\"CB\",\"type\":\"input\"},{\"id\":\"ClntH\",\"label\":\"CH\",\"type\":\"foundation.thermal.thermal\"},{\"id\":\"AmbH\",\"label\":\"AH\",\"type\":\"foundation.thermal.thermal\"}],\"Right\":[],\"Top\":[{\"id\":\"p\",\"label\":\"+\",\"type\":\"foundation.electrical.electrical\"}]}"
  Module1_outputs : SimscapeProbe  BoundBlock=1668  Variables={iCellModel, numCyclesCellModel, socCellModel, socParallelAssembly, temperatureCellModel, vCellModel, vParallelAssembly}
  balancingSelector1 : Selector  InputPortWidth=14  IndexOptions=Index vector (dialog)  Indices="[1   2   3   4   5   6   7   8   9  10  11  12  13  14]"  OutputSizes=1
  iCellModelMux : Mux  Inputs=1
  numCyclesCellModelMux : Mux  Inputs=1
  socCellModelMux : Mux  Inputs=1
  socParallelAssemblyMux : Mux  Inputs=1
  temperatureCellModelMux : Mux  Inputs=1
  vCellModelMux : Mux  Inputs=1
  vParallelAssemblyMux : Mux  Inputs=1
  + : PMIOPort  Side=Left
  - : PMIOPort  Port=2  Side=Right
  AmbH : PMIOPort  Port=3  Side=Right
  ClntH : PMIOPort  Port=4  Side=Right
  iCellModel : Outport
  numCyclesCellModel : Outport  Port=2
  socCellModel : Outport  Port=3
  socParallelAssembly : Outport  Port=4
  temperatureCellModel : Outport  Port=5
  vCellModel : Outport  Port=6
  vParallelAssembly : Outport  Port=7
  wires:
  [balancing1] -> Converter1/1
  balancingSelector1/1 -> [balancing1]
  balancing/1 -> balancingSelector1/1
  [vParallelAssembly1] -> vParallelAssemblyMux/1
  vParallelAssemblyMux/1 -> vParallelAssembly/1
  Module1_outputs/1 -> [iCellModel1]
  [vCellModel1] -> vCellModelMux/1
  vCellModelMux/1 -> vCellModel/1
  Module1_outputs/2 -> [numCyclesCellModel1]
  [temperatureCellModel1] -> temperatureCellModelMux/1
  temperatureCellModelMux/1 -> temperatureCellModel/1
  Module1_outputs/3 -> [socCellModel1]
  [socParallelAssembly1] -> socParallelAssemblyMux/1
  socParallelAssemblyMux/1 -> socParallelAssembly/1
  Module1_outputs/4 -> [socParallelAssembly1]
  [socCellModel1] -> socCellModelMux/1
  socCellModelMux/1 -> socCellModel/1
  Module1_outputs/5 -> [temperatureCellModel1]
  [numCyclesCellModel1] -> numCyclesCellModelMux/1
  numCyclesCellModelMux/1 -> numCyclesCellModel/1
  Module1_outputs/6 -> [vCellModel1]
  [iCellModel1] -> iCellModelMux/1
  iCellModelMux/1 -> iCellModel/1
  Module1_outputs/7 -> [vParallelAssembly1]
  connections:
  Converter1/RConn1 -- Module1/LConn1
  ClntH_From_1/LConn1 -- ClntH/RConn1
  ClntH_To_1/LConn1 -- Module1/LConn2
  AmbH_From_1/LConn1 -- AmbH/RConn1
  AmbH_To_1/LConn1 -- Module1/LConn3
  Module1/RConn1 -- -/RConn1
  Module1/LConn4 -- +/RConn1

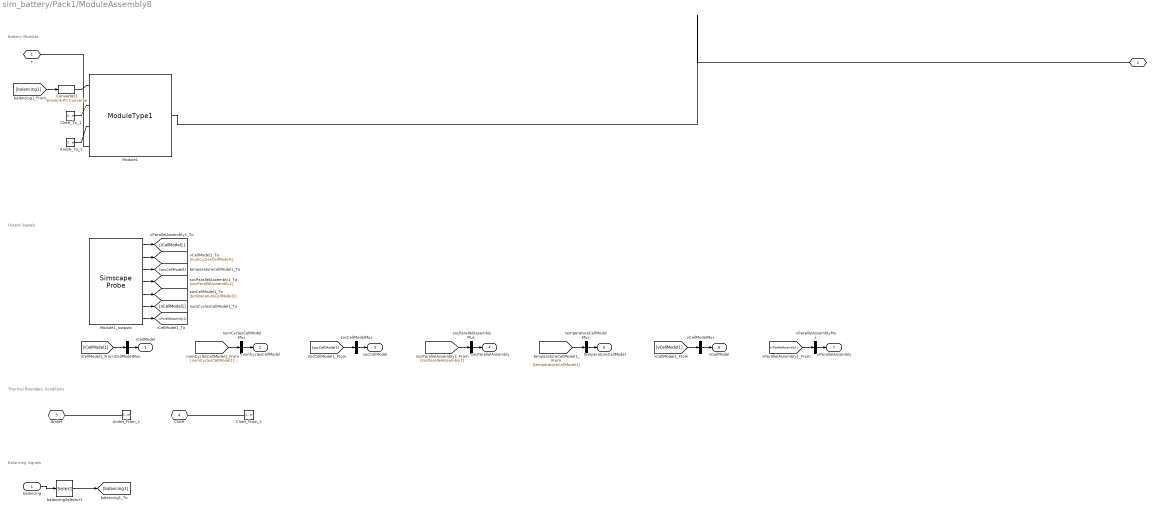
== system sim_battery/Pack1/ModuleAssembly8 ==
  note: Balancing Signals
  note: Thermal Boundary Conditions
  note: Output Signals
  note: Battery Modules
  balancing : Inport  PortDimensions=14
  AmbH_From_1 : ConnectionLabel  Label=ambH_1
  AmbH_To_1 : ConnectionLabel  Label=ambH_1
  ClntH_From_1 : ConnectionLabel  Label=clntH_1
  ClntH_To_1 : ConnectionLabel  Label=clntH_1
  Converter1 : nesl_utility/Simulink-PS Converter  PhysicalDomain=network_engine_domain  SubClassName=ps_input  LeftPortType=input  RightPortType=output  PseudoPeriodic=off  Frequencies=[]  NoiseDistribution=none  NoiseParameters=[]  Unit=1  AffineConversion=off  FilteringAndDerivatives=provide  SimscapeFilterOrder=1  InputFilterTimeConstant=0.001  UdotUserProvided=0
  Module1 : GD_Batterymodel_5_lib/Modules/ModuleType1  SOC_vec=ModuleType1.SOC_vec  T_vec=ModuleType1.T_vec K  V0_mat=ModuleType1.V0_mat V  V_range=ModuleType1.V_range V  R0_mat=ModuleType1.R0_mat Ohm  AH=ModuleType1.AH A*hr  extrapolation_option=simscape.enum.extrapolation.nearest  R1_mat=ModuleType1.R1_mat Ohm  tau1_mat=ModuleType1.tau1_mat s  R2_mat=ModuleType1.R2_mat Ohm  tau2_mat=ModuleType1.tau2_mat s  thermal_mass=ModuleType1.thermal_mass J/K  CoolantResistance=ModuleType1.CoolantResistance K/W  AmbientResistance=ModuleType1.AmbientResistance K/W  CellBalancingClosedResistance=ModuleType1.CellBalancingClosedResistance Ohm  CellBalancingOpenConductance=ModuleType1.CellBalancingOpenConductance 1/Ohm  CellBalancingThreshold=ModuleType1.CellBalancingThreshold  CellBalancingResistance=ModuleType1.CellBalancingResistance Ohm  P=3  S=14  iCellModel_specify=on  iCellModel_priority=None  iCellModel=ModuleAssembly8.Module1.iCellModel A  iCellModel_nominal_specify=off  iCellModel_nominal_unit=A  iCellModel_nominal_value=1  vCellModel_specify=on  vCellModel_priority=None  vCellModel=ModuleAssembly8.Module1.vCellModel V  vCellModel_nominal_specify=off  vCellModel_nominal_unit=V  vCellModel_nominal_value=1  socCellModel_specify=on  socCellModel_priority=High  socCellModel=ModuleAssembly8.Module1.socCellModel  socCellModel_nominal_specify=off  socCellModel_nominal_unit=1  socCellModel_nominal_value=1  numCyclesCellModel_specify=on  numCyclesCellModel_priority=High  numCyclesCellModel=ModuleAssembly8.Module1.numCyclesCellModel  numCyclesCellModel_nominal_specify=off  numCyclesCellModel_nominal_unit=1  numCyclesCellModel_nominal_value=1  temperatureCellModel_specify=on  temperatureCellModel_priority=High  temperatureCellModel=ModuleAssembly8.Module1.temperatureCellModel K  temperatureCellModel_nominal_specify=off  temperatureCellModel_nominal_unit=K  temperatureCellModel_nominal_value=1  vParallelAssembly_specify=on  vParallelAssembly_priority=None  vParallelAssembly=ModuleAssembly8.Module1.vParallelAssembly V  vParallelAssembly_nominal_specify=off  vParallelAssembly_nominal_unit=V  vParallelAssembly_nominal_value=1  socParallelAssembly_specify=on  socParallelAssembly_priority=None  socParallelAssembly=ModuleAssembly8.Module1.socParallelAssembly  socParallelAssembly_nominal_specify=off  socParallelAssembly_nominal_unit=1  socParallelAssembly_nominal_value=1
      settings: InternalSimscapePortConfiguration="{\"Bottom\":[{\"id\":\"n\",\"label\":\"-\",\"type\":\"foundation.electrical.electrical\"}],\"Left\":[{\"id\":\"enableCellBalancing\",\"label\":\"CB\",\"type\":\"input\"},{\"id\":\"ClntH\",\"label\":\"CH\",\"type\":\"foundation.thermal.thermal\"},{\"id\":\"AmbH\",\"label\":\"AH\",\"type\":\"foundation.thermal.thermal\"}],\"Right\":[],\"Top\":[{\"id\":\"p\",\"label\":\"+\",\"type\":\"foundation.electrical.electrical\"}]}"
  Module1_outputs : SimscapeProbe  BoundBlock=1716  Variables={iCellModel, numCyclesCellModel, socCellModel, socParallelAssembly, temperatureCellModel, vCellModel, vParallelAssembly}
  balancingSelector1 : Selector  InputPortWidth=14  IndexOptions=Index vector (dialog)  Indices="[1   2   3   4   5   6   7   8   9  10  11  12  13  14]"  OutputSizes=1
  iCellModelMux : Mux  Inputs=1
  numCyclesCellModelMux : Mux  Inputs=1
  socCellModelMux : Mux  Inputs=1
  socParallelAssemblyMux : Mux  Inputs=1
  temperatureCellModelMux : Mux  Inputs=1
  vCellModelMux : Mux  Inputs=1
  vParallelAssemblyMux : Mux  Inputs=1
  + : PMIOPort  Side=Left
  - : PMIOPort  Port=2  Side=Right
  AmbH : PMIOPort  Port=3  Side=Right
  ClntH : PMIOPort  Port=4  Side=Right
  iCellModel : Outport
  numCyclesCellModel : Outport  Port=2
  socCellModel : Outport  Port=3
  socParallelAssembly : Outport  Port=4
  temperatureCellModel : Outport  Port=5
  vCellModel : Outport  Port=6
  vParallelAssembly : Outport  Port=7
  wires:
  [balancing1] -> Converter1/1
  balancingSelector1/1 -> [balancing1]
  balancing/1 -> balancingSelector1/1
  [vParallelAssembly1] -> vParallelAssemblyMux/1
  vParallelAssemblyMux/1 -> vParallelAssembly/1
  Module1_outputs/1 -> [iCellModel1]
  [vCellModel1] -> vCellModelMux/1
  vCellModelMux/1 -> vCellModel/1
  Module1_outputs/2 -> [numCyclesCellModel1]
  [temperatureCellModel1] -> temperatureCellModelMux/1
  temperatureCellModelMux/1 -> temperatureCellModel/1
  Module1_outputs/3 -> [socCellModel1]
  [socParallelAssembly1] -> socParallelAssemblyMux/1
  socParallelAssemblyMux/1 -> socParallelAssembly/1
  Module1_outputs/4 -> [socParallelAssembly1]
  [socCellModel1] -> socCellModelMux/1
  socCellModelMux/1 -> socCellModel/1
  Module1_outputs/5 -> [temperatureCellModel1]
  [numCyclesCellModel1] -> numCyclesCellModelMux/1
  numCyclesCellModelMux/1 -> numCyclesCellModel/1
  Module1_outputs/6 -> [vCellModel1]
  [iCellModel1] -> iCellModelMux/1
  iCellModelMux/1 -> iCellModel/1
  Module1_outputs/7 -> [vParallelAssembly1]
  connections:
  Converter1/RConn1 -- Module1/LConn1
  ClntH_From_1/LConn1 -- ClntH/RConn1
  ClntH_To_1/LConn1 -- Module1/LConn2
  AmbH_From_1/LConn1 -- AmbH/RConn1
  AmbH_To_1/LConn1 -- Module1/LConn3
  Module1/RConn1 -- -/RConn1
  Module1/LConn4 -- +/RConn1
